simulink model "blackbanana_kincon_ver2"  (R2022b)
settings: Solver=VariableStepAuto  StartTime=0.0  StopTime=20  RelTol=1e-3
undefined symbols (not defined in the file): kinesis_efos, kinesis_ondemand, kinesis_peak, kinesis_records
settings Model: Creator=KarlO  LastModifiedBy=KarlO

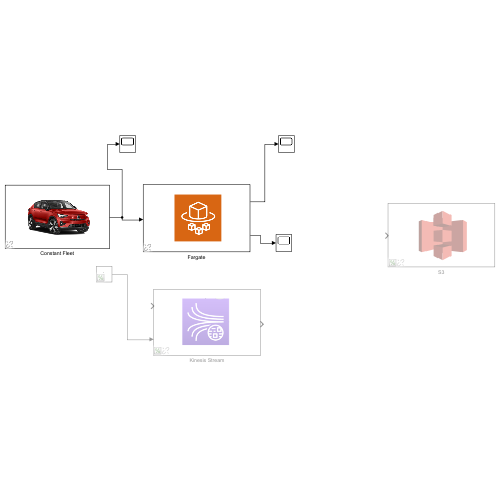
[thumbnail: Simulink's stored preview of the top-level diagram]
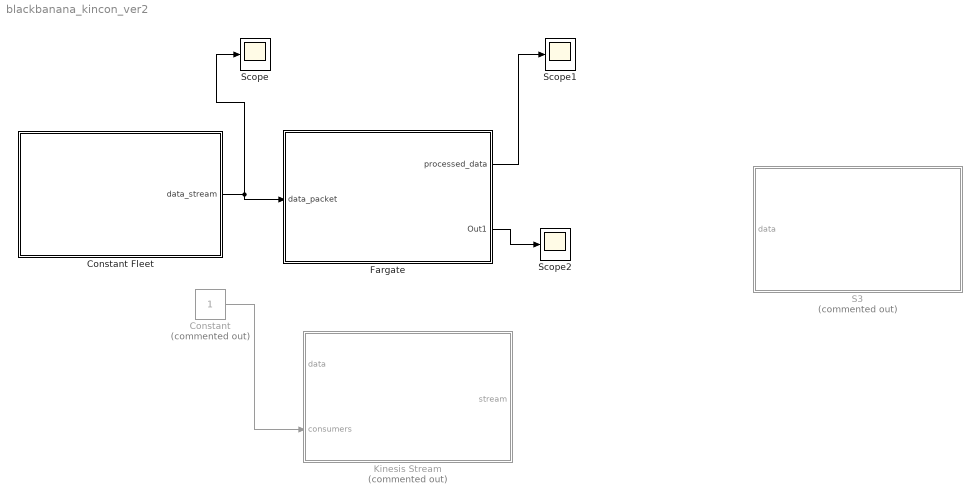
== system blackbanana_kincon_ver2 ==
  Constant : Constant  Commented=on
  Constant Fleet : Subsystem  AncestorBlock=VACLib/Vehicle Components/Constant Fleet
      settings: LibrarySourceBlock=VACLib/Vehicle Components/Constant Fleet
      mask Display: image('C:\Users\KarlO\architectural-tradeoff-analysis\DCA-simulator\Volvo Architecture\VAC library\Images\VAC\cc9459c7a9e4acd4eb37509497aa20bf.png',[40,10,125,100]); % Use "Edit Image" on toolstrip to change.
  Fargate : Subsystem  AncestorBlock=VACLib/AWS Components/Fargate
      settings: LibrarySourceBlock=VACLib/AWS Components/Fargate
      mask Display: image('C:\Users\KarlO\architectural-tradeoff-analysis\DCA-simulator\Volvo Architecture\VAC library\Images\VAC\fargate.png',[60,20,90,90]); % Use "Edit Image" on toolstrip to change.
  Kinesis Stream : Subsystem  Commented=on  AncestorBlock=VACLib/AWS Components/Kinesis Stream
      settings: LibrarySourceBlock=VACLib/AWS Components/Kinesis Stream
      mask Display: image('C:\Users\KarlO\architectural-tradeoff-analysis\DCA-simulator\Volvo Architecture\VAC library\Images\VAC\kinesis2.png',[55,20,90,90]); % Use "Edit Image" on toolstrip to change.
  S3 : Subsystem  Commented=on  AncestorBlock=VACLib/AWS Components/S3
      settings: LibrarySourceBlock=VACLib/AWS Components/S3
      mask Display: image('C:\Users\KarlO\architectural-tradeoff-analysis\DCA-simulator\Volvo Architecture\VAC library\Images\VAC\Amazon-S3-Logo.svg',[55,10,100,100]); % Use "Edit Image" on toolstrip to change.
  Scope : Scope
  Scope1 : Scope
  Scope2 : Scope
  wires:
  Constant/1 -> Kinesis Stream/2(consumers)
  Constant Fleet/1(data_stream) -> Scope/1, Fargate/1(data_packet)
  Fargate/1(processed_data) -> Scope1/1
  Fargate/2(Out1) -> Scope2/1

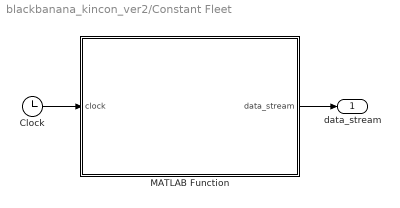
== system blackbanana_kincon_ver2/Constant Fleet ==
  Clock : Clock
  MATLAB Function : MATLAB Function  TreatAsAtomicUnit=on
  data_stream : Outport
  wires:
  Clock/1 -> MATLAB Function/1(clock)
  MATLAB Function/1(data_stream) -> data_stream/1

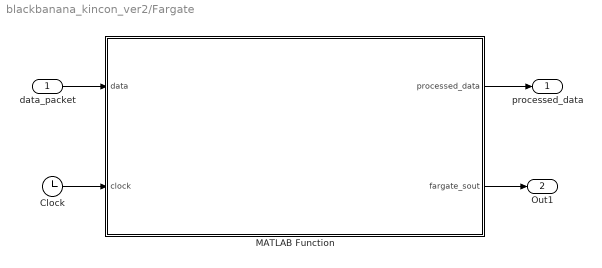
== system blackbanana_kincon_ver2/Fargate ==
  data_packet : Inport
  Clock : Clock
  MATLAB Function : MATLAB Function  TreatAsAtomicUnit=on
  processed_data : Outport
  Out1 : Outport  Port=2
  wires:
  MATLAB Function/2(fargate_sout) -> Out1/1
  MATLAB Function/1(processed_data) -> processed_data/1
  data_packet/1 -> MATLAB Function/1(data)
  Clock/1 -> MATLAB Function/2(clock)

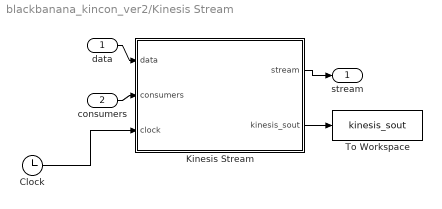
== system blackbanana_kincon_ver2/Kinesis Stream ==
  data : Inport
  consumers : Inport  Port=2
  Clock : Clock
  Kinesis Stream : MATLAB Function  TreatAsAtomicUnit=on
  To Workspace : ToWorkspace  VariableName=kinesis_sout  SaveFormat=Timeseries  SampleTime=-1
  stream : Outport
  wires:
  Kinesis Stream/2(kinesis_sout) -> To Workspace/1
  Clock/1 -> Kinesis Stream/3(clock)
  consumers/1 -> Kinesis Stream/2(consumers)
  Kinesis Stream/1(stream) -> stream/1
  data/1 -> Kinesis Stream/1(data)

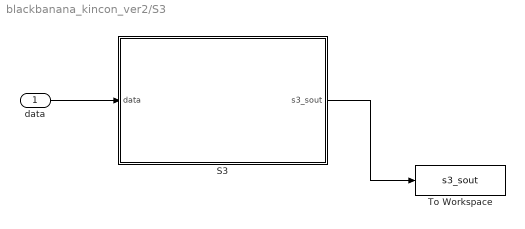
== system blackbanana_kincon_ver2/S3 ==
  data : Inport
  S3 : MATLAB Function  TreatAsAtomicUnit=on
  To Workspace : ToWorkspace  VariableName=s3_sout  SaveFormat=Timeseries  SampleTime=-1
  wires:
  data/1 -> S3/1(data)
  S3/1(s3_sout) -> To Workspace/1

== matlab function blackbanana_kincon_ver2/Constant Fleet/MATLAB Function ==
  data: clock input; data_stream output
function data_stream  = fcn(clock)

persistent out;
persistent last_tick;
persistent data_to_send;

message_size = 1;
car_cache = 2;
fleet_size = 1000;
simulation_time = 10;

if isempty(out)
    out = 0;
    data_to_send = (message_size*fleet_size*simulation_time);
    last_tick = 0;
end

tick = clock;
passed_time = tick-last_tick;
last_tick = tick;

send_this_tick = (data_to_send/simulation_time)*passed_time;

to_send = floor(send_this_tick/(car_cache*message_size));

if tick >= simulation_time
    out = data_to_send;
else
    out = out + (to_send*car_cache*message_size);
end

data_stream = [out,(car_cache*message_size), fleet_size, simulation_time];

== matlab function blackbanana_kincon_ver2/Fargate/MATLAB Function ==
  data: processed_data output; data input; fargate_sout output; clock input
function [processed_data,fargate_sout] = fargate(data, clock)

persistent computed_data;
persistent received_data;
persistent elapsed_time;
persistent active_tasks;
persistent remaining_comptasks;
persistent accumulated_latency;
persistent cost;
persistent memory;

fargate_vcpus = 4;
fargate_memorylevel = 3;

if isempty(computed_data)
    computed_data = 0;
    received_data = 0;
    elapsed_time = 0;
    active_tasks = 1;
    remaining_comptasks = 0;
    accumulated_latency = 0;
    cost = 0;
    memory = (fargate_vcpus * 2 * fargate_memorylevel);
end

new_data = data(1) - received_data;
chunk_size = data(2);
%fleet_size = data(3);
%simulation_time = data(4);

%maaaagic
comptasks_per_second = fargate_vcpus * fargate_memorylevel * 200;


if new_data > 0 || remaining_comptasks > 0
    tick = clock - elapsed_time;
    elapsed_time = clock;
    received_data = received_data + new_data;

    remaining_comptasks = remaining_comptasks + floor(new_data/chunk_size);

    tasks_needed = floor(remaining_comptasks/(comptasks_per_second*tick));

    if tasks_needed == 0
        active_tasks = 1;
    else
        delta = max(tasks_needed-active_tasks,0);
        accumulated_latency = accumulated_latency + (delta*60);
        active_tasks = tasks_needed;
    end
    
    remaining_comptasks = max(remaining_comptasks - (active_tasks*comptasks_per_second*tick),0);

    cpu_cost = active_tasks * fargate_vcpus * (0.04048/3600)* tick;
    memory_cost = active_tasks * memory * (0.004445/3600)* tick;
    cost = cost + (cpu_cost + memory_cost);

end

processed_messages = received_data/(0.008*chunk_size);
latency = accumulated_latency / processed_messages;

fargate_sout = [cost,latency,0,0];
processed_data = [data(1),data(2),data(3),data(4)];

== matlab function blackbanana_kincon_ver2/S3/S3 ==
  data: data input; s3_sout output
function s3_sout = S3(data)

% Keeps count of amount of data buckets (MB)
persistent in_storage;
% Overall cost for usage
persistent s3_cost;

if isempty(in_storage)
    in_storage = 0;
    s3_cost = 0;
end

% Received data (Might be zero if read in between pulses)
% data_packets = (size_sent_in_total, size_of_each_file)
new_data = max(0,data(1) - in_storage);
in_storage = in_storage + new_data;
chunk_size = data(2);

if (new_data > 0)
    % Count packets
    no_of_packets = chunk_size/new_data;
    % Upfront cost ($0.005 per 1000 PUT)
    s3_cost = s3_cost + no_of_packets*0.000005;
end

% [latency, cost, reliability, scalability]
s3_sout = [0, s3_cost,0,0];

== matlab function blackbanana_kincon_ver2/Kinesis Stream/Kinesis Stream ==
  data: data input; stream output; consumers input; kinesis_sout output; clock input; kinesis_ondemand parameter; kinesis_efos parameter; kinesis_records parameter; kinesis_peak parameter
function [stream, kinesis_sout] = kinesis(data, consumers, clock, kinesis_ondemand, kinesis_efos, kinesis_records, kinesis_peak)

persistent received_data;
persistent accepted_data;
persistent streamed_data;
persistent time_passed;
persistent last_received;
persistent running_time;
persistent peak_buffer;
persistent peak_records;

if isempty(received_data)
    received_data = 0;
    accepted_data = 0;
    streamed_data = 0;
    time_passed = 0;
    last_received = 0;
    running_time = 0;
    peak_records = kinesis_records*(1+kinesis_peak);
    peak_buffer = max(0, kinesis_peak);
end

% Get delta data
new_data = max(0,data(1) - received_data);

record_size = data(2);

if(kinesis_ondemand)
    if new_data > 0
        time_passed = clock-last_received;
        running_time = running_time + time_passed;
        last_received = clock;
        received_data = received_data + new_data;

        data_not_accepted = received_data - accepted_data;
        accepted_data = accepted_data + data_not_accepted;

        data_not_streamed = accepted_data - streamed_data;
        data_to_stream = min(data_not_streamed,...
            round(kinesis_efos*2*time_passed));

        streamed_data = streamed_data + data_to_stream;
    end

    data_in_cost = (streamed_data/1000) * 0.08;
    data_out_cost = consumers * (streamed_data/1000) * 0.04;
    stream_cost = (running_time/3600) * 0.04;
    fan_out_cost = kinesis_efos * (streamed_data/1000) * 0.05;

    cost = stream_cost + data_in_cost + data_out_cost + fan_out_cost;
else
    if new_data > 0
        time_passed = clock-last_received;
        running_time = running_time + time_passed;
        last_received = clock;
        received_data = received_data + new_data;

        data_not_accepted = received_data - accepted_data;
        data_to_accept = min(data_not_accepted, ...
            peak_records*record_size*time_passed);
        accepted_data = accepted_data + data_to_accept;

        data_not_streamed = accepted_data - streamed_data;
        data_to_stream = min(data_not_streamed, ...
            round(kinesis_efos*2*peak_records*record_size*time_passed));

        streamed_data = streamed_data + data_to_stream;
    end

    b = peak_records*record_size;
    c = peak_records*record_size*consumers*0.5;
    d = peak_records/1000;
    a = max(b,c);
    a = max(a,d);
    a = max(a,1);

    shards_needed = round(a);
    shards_needed = round(shards_needed + shards_needed*(peak_buffer/100));
    
    put_payload_units = round(record_size/25);

    base_size = (kinesis_records * record_size * running_time)/1000;

    shard_hours_cost = shards_needed * running_time * 0.015;
    payload_units_cost = put_payload_units * ...
        kinesis_records * running_time * 0.000000014;
    efo_consumers_shard_hours_cost = shards_needed * (running_time/3600)...
        * kinesis_efos * 0.015 ; 
    efo_data_retrievals_cost = kinesis_efos * base_size * 0.013;

    cost = shard_hours_cost + payload_units_cost + ...
        efo_data_retrievals_cost + efo_consumers_shard_hours_cost;
end

kinesis_sout = [0,cost,0,0];
stream = [data(1),data(2),data(3),data(4)];
